simulink model "test_proof"  (Simulink 8.7)
settings: Solver=FixedStepDiscrete  StartTime=0.0  StopTime=10.0  FixedStep=0.01  RelTol=1e-3
undefined symbols (not defined in the file): PROOF, SETUP
libraries: sldvlib x2
settings DataIOCC: LimitDataPoints=off  SaveFormat=Dataset
settings DebuggingCC: UnderspecifiedInitializationDetection=Simplified  MergeDetectMultiDrivingBlocksExec=error
settings HardwareCC: ProdBitPerPointer=64  ProdLargestAtomicFloat=Float  ProdIntDivRoundTo=Zero  ProdEndianess=LittleEndian  ProdWordSize=64  ProdHWDeviceType=Intel->x86-64 (Windows64)
settings ModelReferenceCC: PropagateSignalLabelsOutOfModel=on
settings ConfigComp: CovModelRefEnable=off  DVTestSuiteOptimization=CombinedObjectives (Nonlinear Extended)  DVSaveHarnessModel=on  DVSaveReport=on  DVReportIncludeGraphics=on

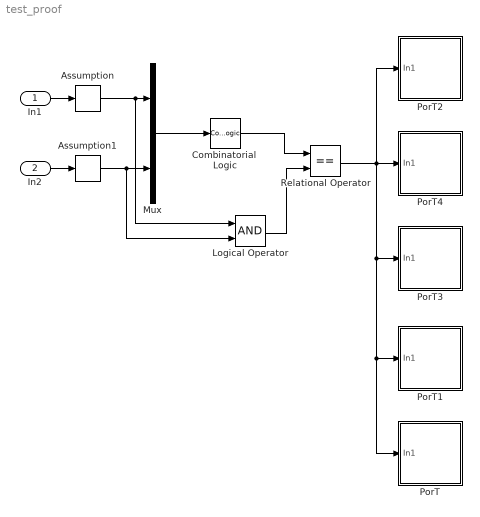
== system test_proof ==
  In1 : Inport
  In2 : Inport  Port=2
  Assumption : sldvlib/Objectives and Constraints/Assumption  enabled=on  customAVTBlockType=Test Condition  intervals={0, 1}  initial=off  dispValues=on  outEnabled=on
      settings: AttributesFormatString=%<intervals>
  Assumption1 : sldvlib/Objectives and Constraints/Assumption  enabled=on  customAVTBlockType=Test Condition  intervals={0, 1}  initial=off  dispValues=on  outEnabled=on
      settings: AttributesFormatString=%<intervals>
  Combinatorial  Logic : CombinatorialLogic  TruthTable=[0;0;0;1]
  Logical Operator : Logic  AllPortsSameDT=off  OutDataTypeStr=boolean
  Mux : Mux  Inputs=2
  PorT : Subsystem  mask(Proof or Test){proof=PROOF, a=on, b=off, c=Trace HL_number, LL_number (Text ..) rfrf, simx=SETUP}
      mask prompts: proof "Proof or Test (0 - Test, 1 - Proof, ELSE use checkbox)"; a "Test"; b "Proof"; c "Requirements"; simx "Setup or Sim (1 - Setup, 0 - Sim)"
      mask help: This block enables the user to set Proof or Test for the Simulink Design Verifier from the Matlab command prompt. With SETUP = 0 the edit postion of the requirements and the check boxes are disabled.
      mask init:
      | if proof == 1
      |     temp=get_param(gcb,'MaskValues');
      |     temp{2}='off';
      |     temp{3}='on';
      |     set_param(gcb,'MaskValues',temp);
      | elseif proof == 0
      |     temp=get_param(gcb,'MaskValues');
      |     temp{2}='on';
      |     temp{3}='off'; 
      |     set_param(gcb,'MaskValues',temp);
      | end
      | if simx==0
      |     set_param(gcb,'MaskEnables',{'on';'off';'off';'off';'on'})
      | else
      |     set_param(gcb,'MaskEnables',{'on';'on';'on';'on';'on'})
      | end
      | proofortest('init',a,b,c,proof,simx)
      mask Display:
      | if (proof == 0) | (a == 1 & b == 0)
      | disp('T')
      | elseif (proof == 1) | (a == 0 & b == 1)
      | disp('P')
      | else
      | disp('Mistake')
      | end
  PorT1 : Subsystem  mask(Proof or Test){proof=PROOF, a=on, b=off, c=Trace HL_number, LL_number (Text ..), simx=SETUP}
      mask prompts: proof "Proof or Test (0 - Test, 1 - Proof, ELSE use checkbox)"; a "Test"; b "Proof"; c "Requirements"; simx "Setup or Sim (1 - Setup, 0 - Sim)"
      mask help: This block enables the user to set Proof or Test for the Simulink Design Verifier from the Matlab command prompt. With SETUP = 0 the edit postion of the requirements and the check boxes are disabled.
      mask init: same as test_proof/PorT
      mask Display:
      | if (proof == 0) | (a == 1 & b == 0)
      | disp('T')
      | elseif (proof == 1) | (a == 0 & b == 1)
      | disp('P')
      | else
      | disp('Mistake')
      | end
  PorT2 : Subsystem  mask(Proof or Test){proof=PROOF, a=on, b=off, c=Trace HL-272727, HL_288282, LL_67373, simx=SETUP}
      mask prompts: proof "Proof or Test (0 - Test, 1 - Proof, ELSE use checkbox)"; a "Test"; b "Proof"; c "Requirements"; simx "Setup or Sim (1 - Setup, 0 - Sim)"
      mask help: This block enables the user to set Proof or Test for the Simulink Design Verifier from the Matlab command prompt. With SETUP = 0 the edit postion of the requirements and the check boxes are disabled.
      mask init: same as test_proof/PorT
      mask Display:
      | if (proof == 0) | (a == 1 & b == 0)
      | disp('T')
      | elseif (proof == 1) | (a == 0 & b == 1)
      | disp('P')
      | else
      | disp('Mistake')
      | end
  PorT3 : Subsystem  mask(Proof or Test){proof=PROOF, a=on, b=off, c=HL_773737, HL_884848, simx=SETUP}
      mask prompts: proof "Proof or Test (0 - Test, 1 - Proof, ELSE use checkbox)"; a "Test"; b "Proof"; c "Requirements"; simx "Setup or Sim (1 - Setup, 0 - Sim)"
      mask help: This block enables the user to set Proof or Test for the Simulink Design Verifier from the Matlab command prompt. With SETUP = 0 the edit postion of the requirements and the check boxes are disabled.
      mask init: same as test_proof/PorT
      mask Display:
      | if (proof == 0) | (a == 1 & b == 0)
      | disp('T')
      | elseif (proof == 1) | (a == 0 & b == 1)
      | disp('P')
      | else
      | disp('Mistake')
      | end
  PorT4 : Subsystem  mask(Proof or Test){proof=PROOF, a=on, b=off, c=Trace HL-272727, HL_288282, simx=SETUP}
      mask prompts: proof "Proof or Test (0 - Test, 1 - Proof, ELSE use checkbox)"; a "Test"; b "Proof"; c "Requirements"; simx "Setup or Sim (1 - Setup, 0 - Sim)"
      mask help: This block enables the user to set Proof or Test for the Simulink Design Verifier from the Matlab command prompt. With SETUP = 0 the edit postion of the requirements and the check boxes are disabled.
      mask init: same as test_proof/PorT
      mask Display:
      | if (proof == 0) | (a == 1 & b == 0)
      | disp('T')
      | elseif (proof == 1) | (a == 0 & b == 1)
      | disp('P')
      | else
      | disp('Mistake')
      | end
  Relational Operator : RelationalOperator  Operator===  OutDataTypeStr=boolean
  wires:
  In1/1 -> Assumption/1
  Mux/1 -> Combinatorial  Logic/1
  In2/1 -> Assumption1/1
  Combinatorial  Logic/1 -> Relational Operator/1
  Logical Operator/1 -> Relational Operator/2
  Relational Operator/1 -> PorT2/1(In1), PorT/1(In1), PorT1/1(In1), PorT3/1(In1), PorT4/1(In1)
  Assumption1/1 -> Logical Operator/2, Mux/2
  Assumption/1 -> Logical Operator/1, Mux/1

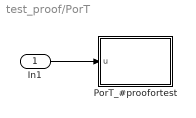
== system test_proof/PorT ==
  In1 : Inport
  PorT_#proofortest : MATLAB Function  TreatAsAtomicUnit=on
      settings: CopyFcn="set_param(gcb, 'Name',  '#proofortest')"
  wires:
  In1/1 -> PorT_#proofortest/1(u)

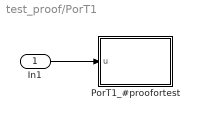
== system test_proof/PorT1 ==
  In1 : Inport
  PorT1_#proofortest : MATLAB Function  TreatAsAtomicUnit=on
      settings: CopyFcn="set_param(gcb, 'Name',  '#proofortest')"
  wires:
  In1/1 -> PorT1_#proofortest/1(u)

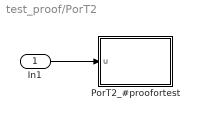
== system test_proof/PorT2 ==
  In1 : Inport
  PorT2_#proofortest : MATLAB Function  TreatAsAtomicUnit=on
      settings: CopyFcn="set_param(gcb, 'Name',  '#proofortest')"
  wires:
  In1/1 -> PorT2_#proofortest/1(u)

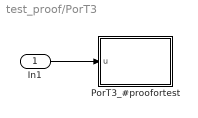
== system test_proof/PorT3 ==
  In1 : Inport
  PorT3_#proofortest : MATLAB Function  TreatAsAtomicUnit=on
      settings: CopyFcn="set_param(gcb, 'Name',  '#proofortest')"
  wires:
  In1/1 -> PorT3_#proofortest/1(u)

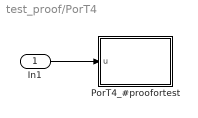
== system test_proof/PorT4 ==
  In1 : Inport
  PorT4_#proofortest : MATLAB Function  TreatAsAtomicUnit=on
      settings: CopyFcn="set_param(gcb, 'Name',  '#proofortest')"
  wires:
  In1/1 -> PorT4_#proofortest/1(u)

== matlab function PorT3/PorT3_#proofortest ==
  data: u input double
function fcn(u)

 sldv.test(u,'HL_773737, HL_884848');

== matlab function PorT2/PorT2_#proofortest ==
  data: u input double
function fcn(u)

 sldv.test(u,'Trace HL-272727, HL_288282, LL_67373');

== matlab function PorT4/PorT4_#proofortest ==
  data: u input double
function fcn(u)

 sldv.test(u,'Trace HL-272727, HL_288282');

== matlab function PorT/PorT_#proofortest ==
  data: u input double
function fcn(u)

 sldv.test(u,'Trace HL_number, LL_number (Text ..) rfrf');

== matlab function PorT1/PorT1_#proofortest ==
  data: u input double
function fcn(u)

 sldv.test(u,'Trace HL_number, LL_number (Text ..)');
